simulink model "untitled1"  (R2019b)
settings: Solver=VariableStepAuto  StartTime=0.0  StopTime=inf  RelTol=1e-3
libraries: CoderSF_BSW_Libs x3, dspstat3 x2
settings Model: EnablePacing=on  Creator=bayra  LastModifiedBy=bayra

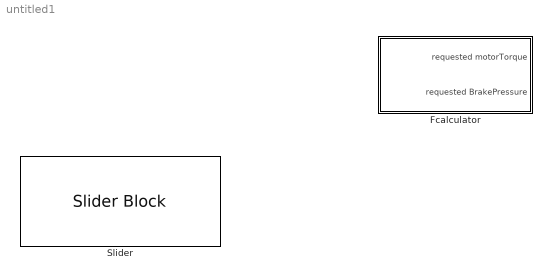
== system untitled1 ==
  "Fcalculator " : Subsystem
  Slider : SliderBlock

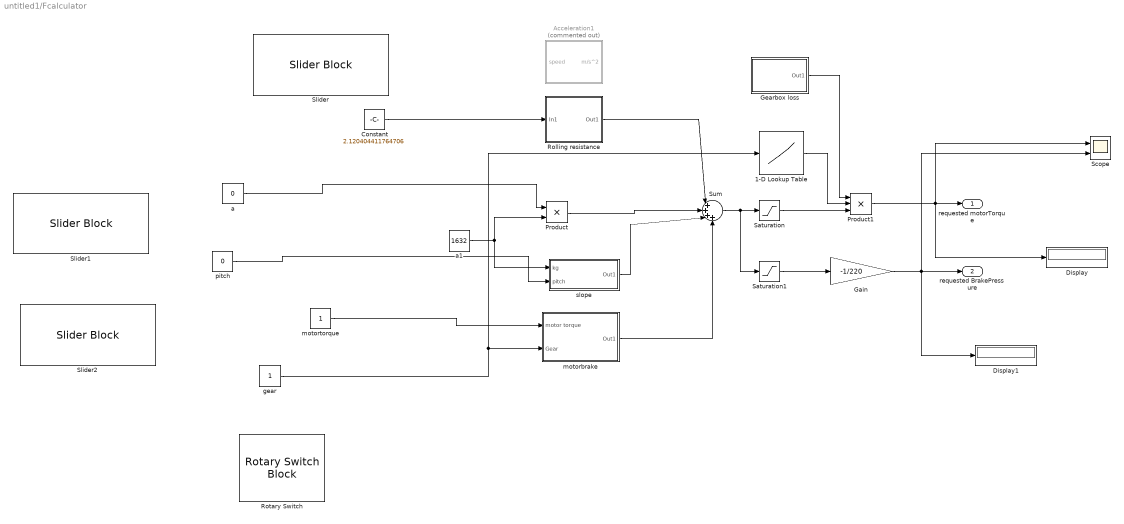
== system untitled1/Fcalculator  ==
  1-D Lookup Table : Lookup_n-D  NumberOfTableDimensions=1  BreakpointsForDimension1=[0 1 2 3 4 5]  Table=[0 1/53.5 1/32.6 1/21.7 1/16.2 1/12.2]  InternalRulePriority=Speed  RndMeth=Simplest  InputSameDT=on
  Acceleration1 : Subsystem  Commented=on
  Constant : Constant  Value=2.120404411764706
  Display : Display
  Display1 : Display
  Gain : Gain  Gain=-1/220
  Gearbox loss : Subsystem
  Product : Product
  Product1 : Product  Inputs=3
  Rolling resistance : Subsystem
  Rotary Switch : RotarySwitchBlock
      settings: Values={{'N', '1', '2', '3', '4', '5'}, [0 1 2 3 4 5]}
  Saturation : Saturate  UpperLimit=3000  LowerLimit=0
  Saturation1 : Saturate  UpperLimit=0  LowerLimit=-10000
  Scope : Scope  NumInputPorts=2
  Slider : SliderBlock  ScaleMax=15
  Slider1 : SliderBlock  ScaleMin=-3  ScaleMax=3
  Slider2 : SliderBlock  ScaleMin=-3  ScaleMax=3
  Sum : Sum  Inputs=|++++
  a : Constant  Value=0
  a1 : Constant  Value=1632
  "gear " : Constant
  motorbrake : Subsystem
  "motortorque " : Constant
  pitch : Constant  Value=0
  slope : Subsystem
  requested motorTorque : Outport
  requested BrakePressure : Outport  Port=2
  wires:
  Constant/1 -> Rolling resistance/1(In1)
  "motortorque "/1 -> motorbrake/1(motor torque)
  Rolling resistance/1(Out1) -> Sum/1
  Product/1 -> Sum/2
  slope/1(Out1) -> Sum/3
  motorbrake/1(Out1) -> Sum/4
  Sum/1 -> Saturation1/1, Saturation/1
  1-D Lookup Table/1 -> Product1/2
  Saturation/1 -> Product1/3
  Gearbox loss/1(Out1) -> Product1/1
  Saturation1/1 -> Gain/1
  Product1/1 -> Display/1, Scope/1, requested motorTorque/1
  a/1 -> Product/1
  a1/1 -> Product/2, slope/1(kg)
  pitch/1 -> slope/2(pitch)
  "gear "/1 -> 1-D Lookup Table/1, motorbrake/2(Gear)
  Gain/1 -> Display1/1, Scope/2, requested BrakePressure/1

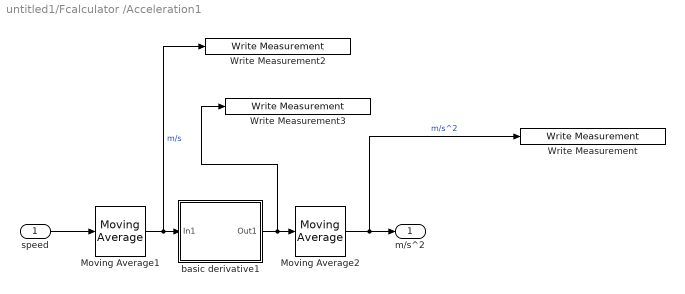
== system untitled1/Fcalculator /Acceleration1 ==
  speed : Inport
  Moving Average1 : dspstat3/Moving Average  Method=Sliding window  ForgettingFactorPort=off  SpecifyWindowLength=on  WindowLength=200  ForgettingFactor=0.9  SimulateUsing=Code generation
  Moving Average2 : dspstat3/Moving Average  Method=Sliding window  ForgettingFactorPort=off  SpecifyWindowLength=on  WindowLength=200  ForgettingFactor=0.9  SimulateUsing=Code generation
  Write Measurement : CoderSF_BSW_Libs/Calibration & Measurement/Write Measurement  variable_name=Golf_ACC_200sample  variable_value=0  variable_type=single  numD=1  unitStr=""  descStr=""
      settings: AttributesFormatString=type:%<variable_type> Dimensions:%<numD>  SourceProductName=EcoCoder Blocks
  Write Measurement2 : CoderSF_BSW_Libs/Calibration & Measurement/Write Measurement  variable_name=debug_Golf_speed_movAvg150sample  variable_value=0  variable_type=single  numD=1  unitStr=ms  descStr=""
      settings: AttributesFormatString=type:%<variable_type> Dimensions:%<numD>  SourceProductName=EcoCoder Blocks
  Write Measurement3 : CoderSF_BSW_Libs/Calibration & Measurement/Write Measurement  variable_name=debug_Golf_ACC150sample  variable_value=0  variable_type=single  numD=1  unitStr=ms2  descStr=""
      settings: AttributesFormatString=type:%<variable_type> Dimensions:%<numD>  SourceProductName=EcoCoder Blocks
  basic derivative1 : Subsystem
  m/s^2 : Outport
  wires:
  Moving Average2/1 -> m/s^2/1, Write Measurement/1  "m/s^2"
  basic derivative1/1(Out1) -> Moving Average2/1, Write Measurement3/1
  speed/1 -> Moving Average1/1
  Moving Average1/1 -> basic derivative1/1(In1), Write Measurement2/1  "m/s"

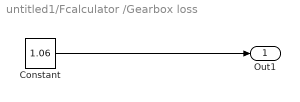
== system untitled1/Fcalculator /Gearbox loss ==
  Constant : Constant  Value=1.06
  Out1 : Outport
  wires:
  Constant/1 -> Out1/1

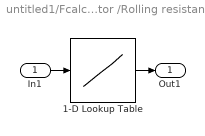
== system untitled1/Fcalculator /Rolling resistance ==
  In1 : Inport
  1-D Lookup Table : Lookup_n-D  NumberOfTableDimensions=1  BreakpointsForDimension1=[0 0.02 8 16]  Table=[0 163.2 228.5 326.4]  InternalRulePriority=Speed  RndMeth=Simplest  InputSameDT=on
  Out1 : Outport
  wires:
  1-D Lookup Table/1 -> Out1/1
  In1/1 -> 1-D Lookup Table/1

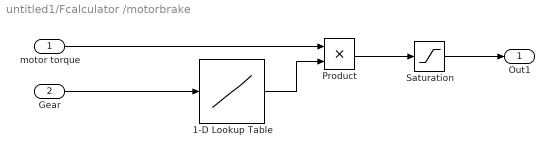
== system untitled1/Fcalculator /motorbrake ==
  motor torque : Inport
  Gear : Inport  Port=2
  1-D Lookup Table : Lookup_n-D  NumberOfTableDimensions=1  BreakpointsForDimension1=[0 1 2 3 4 5]  Table=[0 53.5 32.6 21.7 16.2 12.2]  InternalRulePriority=Speed  RndMeth=Simplest  InputSameDT=on
  Product : Product
  Saturation : Saturate  UpperLimit=0  LowerLimit=-inf
  Out1 : Outport
  wires:
  Gear/1 -> 1-D Lookup Table/1
  1-D Lookup Table/1 -> Product/2
  motor torque/1 -> Product/1
  Product/1 -> Saturation/1
  Saturation/1 -> Out1/1

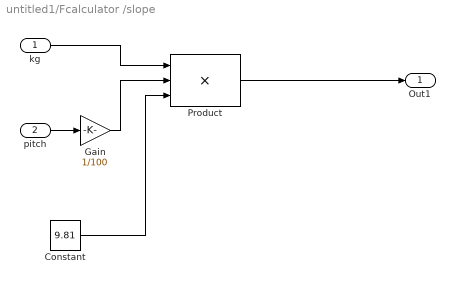
== system untitled1/Fcalculator /slope ==
  kg : Inport
  pitch : Inport  Port=2
  Constant : Constant  Value=9.81
  Gain : Gain  Gain=1/100
  Product : Product  Inputs=3
  Out1 : Outport
  wires:
  kg/1 -> Product/1
  pitch/1 -> Gain/1
  Constant/1 -> Product/3
  Product/1 -> Out1/1
  Gain/1 -> Product/2

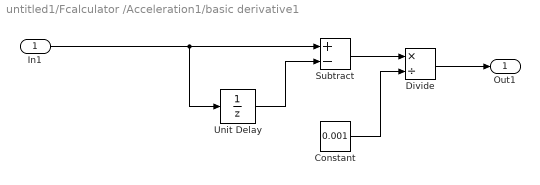
== system untitled1/Fcalculator /Acceleration1/basic derivative1 ==
  In1 : Inport
  Constant : Constant  Value=0.001  OutDataTypeStr=single
  Divide : Product  Inputs=*/
  Subtract : Sum  Inputs=+-
  Unit Delay : UnitDelay  SampleTime=-1  HasFrameUpgradeWarning=on
  Out1 : Outport
  wires:
  Unit Delay/1 -> Subtract/2
  Subtract/1 -> Divide/1
  Constant/1 -> Divide/2
  Divide/1 -> Out1/1
  In1/1 -> Subtract/1, Unit Delay/1
